simulink model "imageSendExample2"  (R2014a)
settings: configuration reference "AR_Drone_ConfigSet" (kept outside this file)
undefined symbols (not defined in the file or in its folder): Afilter, Afilterphi, Amat, Bd, KDphi, KDphi_adjust, KDpsic, KDtheta, KDtheta_adjust, KDxc, KDyc, KDzc, KPphi, KPphi_adjust, KPpsic, KPtheta, KPtheta_adjust, KPxc, KPyc, KPzc, L, LA, LAphi, m
libraries: simulink x8, dspmtrx3 x5, AR_Drone_2_Library x4, dspstat3 x2, ARdrone_video_lib x1
(part 1 of 2)
settings Model: SimulationMode=external  Creator=Catarina  LastModifiedBy=Catarina

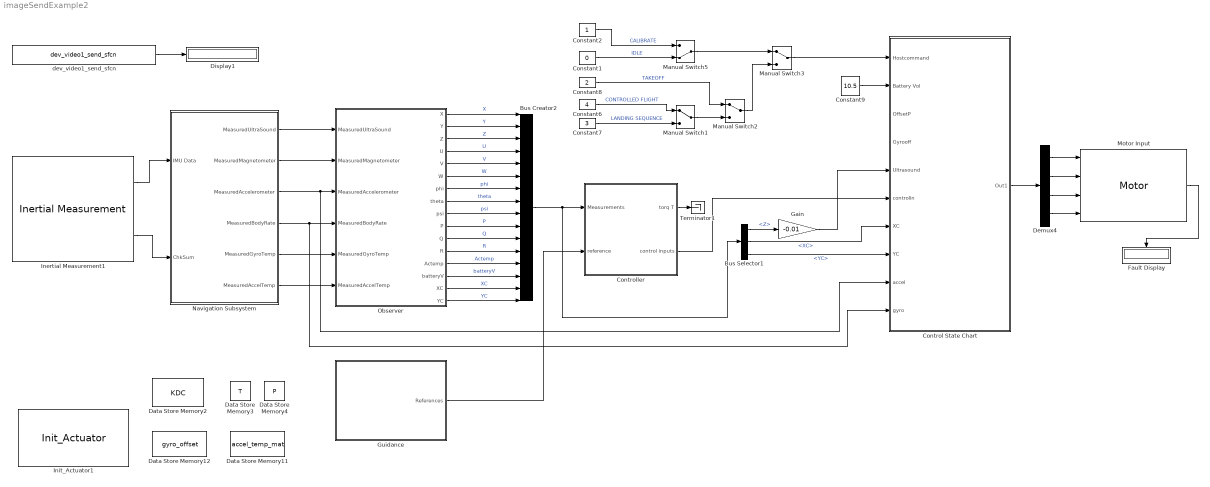
== system imageSendExample2 ==
  Bus Creator2 : BusCreator  Inputs='X','Y','Z','U','V','W','phi','theta','psi','P','Q','R','Actemp','batteryV','XC','YC'
  Bus Selector1 : BusSelector  OutputSignals=Z,XC,YC
  Constant1 : Constant  Value=0
  Constant2 : Constant
  Constant6 : Constant  Value=4
  Constant7 : Constant  Value=3
  Constant8 : Constant  Value=2
  Constant9 : Constant  Value=10.5
  Control State Chart : Subsystem
  Controller : Subsystem
  Data Store Memory11 : DataStoreMemory  DataStoreName=accel_temp_mat  ReadBeforeWriteMsg=warning  WriteAfterWriteMsg=warning  WriteAfterReadMsg=warning  InitialValue=[0 0 0; 0 0 0; 0 0 0]  OutDataTypeStr=double
  Data Store Memory12 : DataStoreMemory  DataStoreName=gyro_offset  ReadBeforeWriteMsg=warning  WriteAfterWriteMsg=warning  WriteAfterReadMsg=warning  InitialValue=[0 0 0]  OutDataTypeStr=double
  Data Store Memory2 : DataStoreMemory  DataStoreName=KDC  ReadBeforeWriteMsg=warning  WriteAfterWriteMsg=warning  WriteAfterReadMsg=warning  OutDataTypeStr=double
  Data Store Memory3 : DataStoreMemory  DataStoreName=T  ReadBeforeWriteMsg=warning  WriteAfterWriteMsg=warning  WriteAfterReadMsg=warning  OutDataTypeStr=double
  Data Store Memory4 : DataStoreMemory  DataStoreName=P  ReadBeforeWriteMsg=warning  WriteAfterWriteMsg=warning  WriteAfterReadMsg=warning  OutDataTypeStr=double
  Demux4 : Demux
  Display1 : Display
  Fault Display : Display
  Gain : Gain  Gain=-0.01
  Guidance : Subsystem
  Inertial Measurement1 : AR_Drone_2_Library/Inertial Measurement  Ts=1/400
  Init_Actuator1 : AR_Drone_2_Library/Init_Actuator  ShowSpec=on
  Manual Switch1 : ManualSwitch
  Manual Switch2 : ManualSwitch
  Manual Switch3 : ManualSwitch
  Manual Switch5 : ManualSwitch  CurrentSetting=0
  Motor Input : AR_Drone_2_Library/Motor
  Navigation Subsystem : Subsystem
  Observer : Subsystem
  Terminator1 : Terminator
  dev_video1_send_sfcn : ARdrone_video_lib/dev_video1_send_sfcn  SFunctionSpec=double y1 = video1GrabSend(int32 work1[1])  SParameter1=[25400]  SParameter2=4  SParameter3=1  SampleTime=1/20  ShowSpec=on
  wires:
  dev_video1_send_sfcn/1 -> Display1/1
  Guidance/1(References) -> Controller/2(reference)
  Constant6/1 -> Manual Switch1/1  "CONTROLLED FLIGHT"
  Constant7/1 -> Manual Switch1/2  "LANDING SEQUENCE"
  Constant8/1 -> Manual Switch2/1  "TAKEOFF"
  Manual Switch1/1 -> Manual Switch2/2
  Constant9/1 -> Control State Chart/2(Battery Vol)
  Controller/2(control inputs) -> Control State Chart/6(controlin)
  Bus Selector1/1 -> Gain/1  "<Z>"
  Bus Selector1/2 -> Control State Chart/7(XC)  "<XC>"
  Bus Selector1/3 -> Control State Chart/8(YC)  "<YC>"
  Gain/1 -> Control State Chart/5(Ultrasound)
  Motor Input/1 -> Fault Display/1
  Demux4/1 -> Motor Input/1
  Demux4/3 -> Motor Input/3
  Control State Chart/1(Out1) -> Demux4/1
  Demux4/4 -> Motor Input/4
  Demux4/2 -> Motor Input/2
  Bus Creator2/1 -> Bus Selector1/1, Controller/1(Measurements)
  Manual Switch2/1 -> Manual Switch3/2
  Inertial Measurement1/1 -> Navigation Subsystem/1(IMU Data)
  Navigation Subsystem/1(MeasuredUltraSound) -> Observer/1(MeasuredUltraSound)
  Navigation Subsystem/2(MeasuredMagnetometer) -> Observer/2(MeasuredMagnetometer)
  Navigation Subsystem/3(MeasuredAccelerometer) -> Control State Chart/9(accel), Observer/3(MeasuredAccelerometer)
  Navigation Subsystem/4(MeasuredBodyRate) -> Control State Chart/10(gyro), Observer/4(MeasuredBodyRate)
  Navigation Subsystem/5(MeasuredGyroTemp) -> Observer/5(MeasuredGyroTemp)
  Navigation Subsystem/6(MeasuredAccelTemp) -> Observer/6(MeasuredAccelTemp)
  Observer/1(X) -> Bus Creator2/1  "X"
  Observer/2(Y) -> Bus Creator2/2  "Y"
  Observer/5(V) -> Bus Creator2/5  "V"
  Observer/4(U) -> Bus Creator2/4  "U"
  Observer/3(Z) -> Bus Creator2/3  "Z"
  Observer/9(psi) -> Bus Creator2/9  "psi"
  Observer/8(theta) -> Bus Creator2/8  "theta"
  Observer/6(W) -> Bus Creator2/6  "W"
  Observer/16(YC) -> Bus Creator2/16  "YC"
  Observer/15(XC) -> Bus Creator2/15  "XC"
  Observer/14(batteryV) -> Bus Creator2/14  "batteryV"
  Observer/13(Actemp) -> Bus Creator2/13  "Actemp"
  Observer/12(R) -> Bus Creator2/12  "R"
  Observer/11(Q) -> Bus Creator2/11  "Q"
  Observer/10(P) -> Bus Creator2/10  "P"
  Observer/7(phi) -> Bus Creator2/7  "phi"
  Manual Switch3/1 -> Control State Chart/1(Hostcommand)
  Constant1/1 -> Manual Switch5/2  "IDLE"
  Constant2/1 -> Manual Switch5/1  "CALIBRATE"
  Manual Switch5/1 -> Manual Switch3/1
  Inertial Measurement1/2 -> Navigation Subsystem/2(ChkSum)
  Controller/1(torq T) -> Terminator1/1

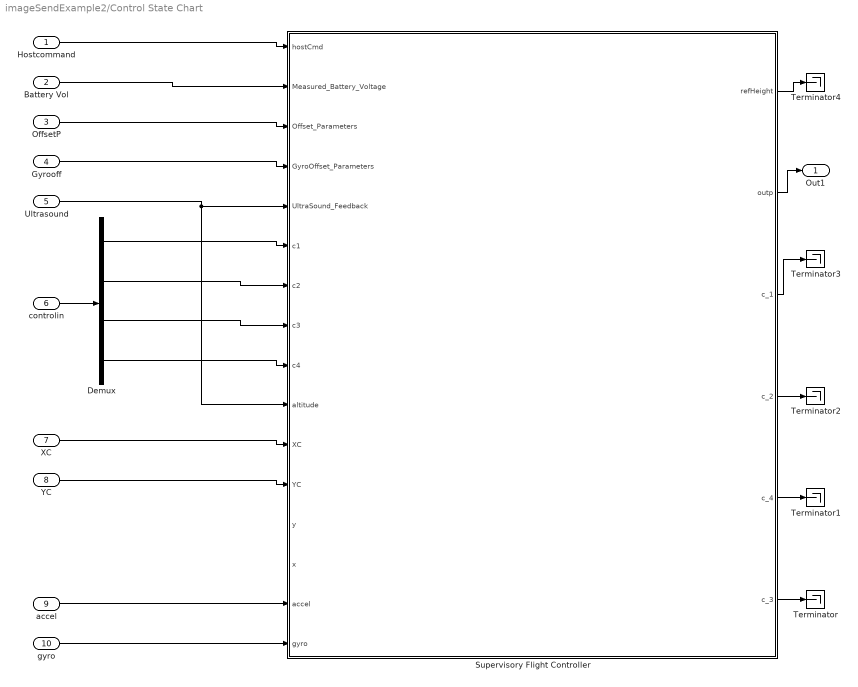
== system imageSendExample2/Control State Chart ==
  Hostcommand : Inport
  Battery Vol : Inport  Port=2
  OffsetP : Inport  Port=3
  Gyrooff : Inport  Port=4
  Ultrasound : Inport  Port=5
  controlin : Inport  Port=6
  XC : Inport  Port=7
  YC : Inport  Port=8
  accel : Inport  Port=9
  gyro : Inport  Port=10
  Demux : Demux
  Supervisory Flight Controller : Stateflow chart  Priority=1  TreatAsAtomicUnit=on
  Terminator{,1..4} (5 alike) : Terminator
  Out1 : Outport
  wires:
  Hostcommand/1 -> Supervisory Flight Controller/1(hostCmd)
  OffsetP/1 -> Supervisory Flight Controller/3(Offset_Parameters)
  Gyrooff/1 -> Supervisory Flight Controller/4(GyroOffset_Parameters)
  Ultrasound/1 -> Supervisory Flight Controller/10(altitude), Supervisory Flight Controller/5(UltraSound_Feedback)
  controlin/1 -> Demux/1
  Battery Vol/1 -> Supervisory Flight Controller/2(Measured_Battery_Voltage)
  Supervisory Flight Controller/2(outp) -> Out1/1
  Demux/1 -> Supervisory Flight Controller/6(c1)
  Demux/2 -> Supervisory Flight Controller/7(c2)
  Demux/3 -> Supervisory Flight Controller/8(c3)
  Demux/4 -> Supervisory Flight Controller/9(c4)
  Supervisory Flight Controller/6(c_3) -> Terminator/1
  Supervisory Flight Controller/3(c_1) -> Terminator3/1
  Supervisory Flight Controller/4(c_2) -> Terminator2/1
  Supervisory Flight Controller/5(c_4) -> Terminator1/1
  Supervisory Flight Controller/1(refHeight) -> Terminator4/1
  XC/1 -> Supervisory Flight Controller/11(XC)
  YC/1 -> Supervisory Flight Controller/12(YC)
  accel/1 -> Supervisory Flight Controller/15(accel)
  gyro/1 -> Supervisory Flight Controller/16(gyro)

== system imageSendExample2/Controller ==
  Measurements : Inport
  reference : Inport  Port=2
  Bus Selector : BusSelector  OutputSignals=X,Y,Z,U,V,W,phi,theta,psi,P,Q,R  OutputAsBus=on
  Control : Subsystem
  Conversion torques to motor speeds : Subsystem
  Mux : Mux
  torq T : Outport
  control inputs : Outport  Port=2
  wires:
  Bus Selector/1 -> Control/1(state)
  Measurements/1 -> Bus Selector/1
  Mux/1 -> Conversion torques to motor speeds/1(torques and thrust), torq T/1
  Control/2(torquephi) -> Mux/2
  Control/3(torquetheta) -> Mux/3
  Control/4(torquepsi) -> Mux/4
  reference/1 -> Control/2(reference)
  Control/1(thrust) -> Mux/1
  Conversion torques to motor speeds/1(Motor speeds) -> control inputs/1

== system imageSendExample2/Guidance ==
  Constant : Constant  Value=0
  Constant1 : Constant  Value=0
  Constant2 : Constant  Value=0
  Data Store Read : DataStoreRead  DataStoreName=KDC
  Gain : Gain  Gain=-1
  Mux2 : Mux  Inputs=16
  References : Outport
  wires:
  Mux2/1 -> References/1
  Constant/1 -> Mux2/9, Mux2/10, Mux2/11, Mux2/12, Mux2/14, Mux2/15, Mux2/16, Mux2/13, Mux2/6, Mux2/5, Mux2/1, Mux2/4
  Constant1/1 -> Mux2/2
  Constant2/1 -> Mux2/8, Mux2/7
  Data Store Read/1 -> Gain/1
  Gain/1 -> Mux2/3

== system imageSendExample2/Navigation Subsystem ==
  IMU Data : Inport
  ChkSum : Inport  Port=2
  CheckSum Pre-Processing : Subsystem
  MeasuredUltraSound : Outport
  MeasuredMagnetometer : Outport  Port=2
  MeasuredAccelerometer : Outport  Port=3
  MeasuredBodyRate : Outport  Port=4
  MeasuredGyroTemp : Outport  Port=5
  MeasuredAccelTemp : Outport  Port=6
  wires:
  IMU Data/1 -> CheckSum Pre-Processing/1(IMU Packets)
  ChkSum/1 -> CheckSum Pre-Processing/2(CheckSumFlag)
  CheckSum Pre-Processing/1(UltraSoundHeight_Processed) -> MeasuredUltraSound/1
  CheckSum Pre-Processing/4(Accelerometer) -> MeasuredAccelerometer/1
  CheckSum Pre-Processing/3(Body Rates - pqr) -> MeasuredBodyRate/1
  CheckSum Pre-Processing/2(Magnetometer_Processed) -> MeasuredMagnetometer/1
  CheckSum Pre-Processing/5(TempMeasure) -> MeasuredGyroTemp/1
  CheckSum Pre-Processing/6(AccelTempMeasure) -> MeasuredAccelTemp/1

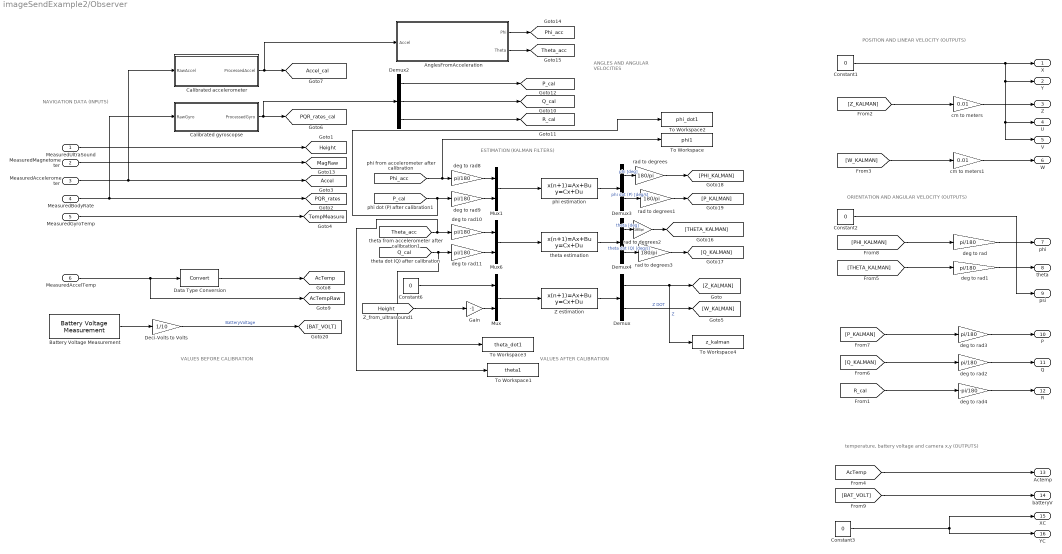
== system imageSendExample2/Observer ==
  note: temperature, battery voltage and camera x,y (OUTPUTS)
  note: ORIENTATION AND ANGULAR VELOCITY (OUTPUTS)
  note: POSITION AND LINEAR VELOCITY (OUTPUTS)
  note: NAVIGATION
      | DATA
      | (INPUTS)
  note: ESTIMATION (KALMAN FILTERS)
  note: ANGLES AND
      | ANGULAR
      | VELOCITIES
  note: VALUES BEFORE CALIBRATION
  note: VALUES AFTER CALIBRATION
  MeasuredUltraSound : Inport
  MeasuredMagnetometer : Inport  Port=2
  MeasuredAccelerometer : Inport  Port=3
  MeasuredBodyRate : Inport  Port=4
  MeasuredGyroTemp : Inport  Port=5
  MeasuredAccelTemp : Inport  Port=6
  AnglesFromAcceleration : Subsystem
  Battery Voltage Measurement : AR_Drone_2_Library/Battery Voltage Measurement  SFunctionSpec=void BatteryMeasure_step(single y1[1])  SampleTime=-1
  Calibrated accelerometer : Subsystem
  Calibrated gyroscopse : Subsystem
  Constant{1..3,6} (4 alike) : Constant  Value=0
  Data Type Conversion : DataTypeConversion
  Deci-Volts to Volts : Gain  Gain=1/10
  Demux : Demux  Outputs=2
  Demux2 : Demux  Outputs=3
  Demux3 : Demux  Outputs=2
  Demux4 : Demux  Outputs=2
  Gain : Gain  Gain=-1
  Mux : Mux  Inputs=2
  Mux1 : Mux  Inputs=2
  Mux6 : Mux  Inputs=2
  To Workspace : ToWorkspace  VariableName=phi1  SaveFormat=Structure With Time  SampleTime=-1
  To Workspace1 : ToWorkspace  VariableName=theta1  SaveFormat=Structure With Time  SampleTime=-1
  To Workspace2 : ToWorkspace  VariableName=phi_dot1  SaveFormat=Structure With Time  SampleTime=-1
  To Workspace3 : ToWorkspace  VariableName=theta_dot1  SaveFormat=Structure With Time  SampleTime=-1
  To Workspace4 : ToWorkspace  VariableName=z_kalman  SaveFormat=Structure With Time  SampleTime=-1
  Z estimation : DiscreteStateSpace  A=Amat  B=[Bd L]  C=eye(2)  D=zeros(2)  X0=[0,0]  SampleTime=-1
  cm to meters : Gain  Gain=0.01
  cm to meters1 : Gain  Gain=0.01
  deg to rad{,1..3,8..11} (8 alike) : Gain  Gain=pi/180
  deg to rad4 : Gain  Gain=-pi/180
  phi estimation : DiscreteStateSpace  A=Afilterphi  B=[LAphi]  C=eye(2)  D=zeros(2)  X0=[0,0]  SampleTime=-1
  rad to degrees{,1..3} (4 alike) : Gain  Gain=180/pi
  theta estimation : DiscreteStateSpace  A=Afilter  B=[LA]  C=eye(2)  D=zeros(2)  X0=[0,0]  SampleTime=-1
  X : Outport
  Y : Outport  Port=2
  Z : Outport  Port=3
  U : Outport  Port=4
  V : Outport  Port=5
  W : Outport  Port=6
  phi : Outport  Port=7
  theta : Outport  Port=8
  psi : Outport  Port=9
  P : Outport  Port=10
  Q : Outport  Port=11
  R : Outport  Port=12
  Actemp : Outport  Port=13
  batteryV : Outport  Port=14
  XC : Outport  Port=15
  YC : Outport  Port=16
  tag scope: AcTemp=global, AcTempRaw=global, Accel=global, Accel_cal=global, Height=global, MagRaw=global, PQR_rates=global, PQR_rates_cal=global, P_cal=global, Phi_acc=global, Q_cal=global, R_cal=global, TempMeasure=global, Theta_acc=global
  wires:
  Mux1/1 -> phi estimation/1
  phi estimation/1 -> Demux3/1
  Battery Voltage Measurement/1 -> Deci-Volts to Volts/1
  MeasuredMagnetometer/1 -> [MagRaw]
  MeasuredAccelerometer/1 -> Calibrated accelerometer/1(RawAccel), [Accel]
  MeasuredGyroTemp/1 -> [TempMeasure]
  MeasuredUltraSound/1 -> [Height]
  Mux6/1 -> theta estimation/1
  theta estimation/1 -> Demux4/1
  Z estimation/1 -> Demux/1
  Constant6/1 -> Mux/1
  Demux/2 -> [W_KALMAN]  "Z DOT"
  Demux/1 -> To Workspace4/1, [Z_KALMAN]  "Z"
  Gain/1 -> Mux/2
  Mux/1 -> Z estimation/1
  [Height] -> Gain/1
  Data Type Conversion/1 -> [AcTemp]
  MeasuredAccelTemp/1 -> [AcTempRaw], Data Type Conversion/1
  Calibrated accelerometer/1(ProcessedAccel) -> [Accel_cal], AnglesFromAcceleration/1(Accel)
  Demux2/2 -> [Q_cal]
  Calibrated gyroscopse/1(ProcessedGyro) -> [PQR_rates_cal], Demux2/1
  Demux2/1 -> [P_cal]
  Demux2/3 -> [R_cal]
  AnglesFromAcceleration/1(Phi) -> [Phi_acc]
  AnglesFromAcceleration/2(Theta) -> [Theta_acc]
  [P_cal] -> To Workspace2/1, deg to rad9/1
  [Q_cal] -> To Workspace3/1, deg to rad11/1
  [Phi_acc] -> To Workspace/1, deg to rad8/1
  Constant1/1 -> V/1, U/1, Y/1, X/1
  [Z_KALMAN] -> cm to meters/1
  [AcTemp] -> Actemp/1
  deg to rad/1 -> phi/1
  cm to meters/1 -> Z/1
  [THETA_KALMAN] -> deg to rad1/1
  [Q_KALMAN] -> deg to rad2/1
  [P_KALMAN] -> deg to rad3/1
  [PHI_KALMAN] -> deg to rad/1
  [BAT_VOLT] -> batteryV/1
  cm to meters1/1 -> W/1
  [W_KALMAN] -> cm to meters1/1
  deg to rad1/1 -> theta/1
  deg to rad3/1 -> P/1
  deg to rad2/1 -> Q/1
  Constant2/1 -> psi/1
  Constant3/1 -> XC/1, YC/1
  Demux4/2 -> rad to degrees3/1  "theta dot (Q) [deg/s]"
  Demux3/1 -> rad to degrees/1  "phi [deg]"
  Demux3/2 -> rad to degrees1/1  "phi dot (P) [deg/s]"
  Demux4/1 -> rad to degrees2/1  "theta [deg]"
  Deci-Volts to Volts/1 -> [BAT_VOLT]  "BatteryVoltage"
  [Theta_acc] -> To Workspace1/1, deg to rad10/1
  deg to rad8/1 -> Mux1/1
  deg to rad9/1 -> Mux1/2
  deg to rad10/1 -> Mux6/1
  deg to rad11/1 -> Mux6/2
  rad to degrees/1 -> [PHI_KALMAN]
  rad to degrees1/1 -> [P_KALMAN]
  rad to degrees2/1 -> [THETA_KALMAN]
  rad to degrees3/1 -> [Q_KALMAN]
  MeasuredBodyRate/1 -> [PQR_rates], Calibrated gyroscopse/1(RawGyro)
  [R_cal] -> deg to rad4/1
  deg to rad4/1 -> R/1

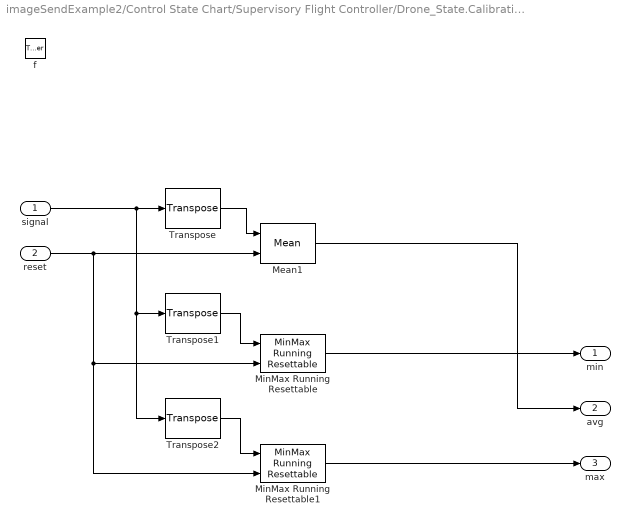
== system imageSendExample2/Control State Chart/Supervisory Flight Controller/Drone_State.Calibration.calibAccel ==
  signal : Inport  OutDataTypeStr=double  PortDimensions=3
  reset : Inport  Port=2  OutDataTypeStr=double  PortDimensions=1
  f : TriggerPort  TriggerType=function-call
      settings: CopyFcn=Stateflow.SLINSF.SimulinkMan.removeBlockPreDeleteFcn  PreDeleteFcn=Stateflow.SLINSF.SimulinkMan.unsafePredeleteFcn
  Mean1 : dspstat3/Mean  run=on  reset_popup=Non-zero sample  InputProcessing=Columns as channels (frame based)  directionMode=Entire input  dimension=1  treatSBRowAsCol=on  roiEnable=off  roiType=Rectangles  roiPortion=Entire ROI  roiOutput=Individual statistics for each ROI  roiFlag=off  outputDataTypeStr=Inherit: Same as accumulator  outputLastDataTypeStr=Inherit: Same as accumulator  outputMin=[]  outputMax=[]  roundingMode=Nearest  overflowMode=off
  MinMax Running Resettable : simulink/Math Operations/MinMax Running Resettable  Function=min  vinit=inf
  MinMax Running Resettable1 : simulink/Math Operations/MinMax Running Resettable  Function=max  vinit=-inf
  Transpose : dspmtrx3/Transpose  Hermitian=off  overflowFlag=off
  Transpose1 : dspmtrx3/Transpose  Hermitian=off  overflowFlag=off
  Transpose2 : dspmtrx3/Transpose  Hermitian=off  overflowFlag=off
  min : Outport
  avg : Outport  Port=2
  max : Outport  Port=3
  wires:
  signal/1 -> Transpose2/1, Transpose1/1, Transpose/1
  Mean1/1 -> avg/1
  Transpose/1 -> Mean1/1
  reset/1 -> MinMax Running Resettable1/2, MinMax Running Resettable/2, Mean1/2
  MinMax Running Resettable1/1 -> max/1
  MinMax Running Resettable/1 -> min/1
  Transpose1/1 -> MinMax Running Resettable/1
  Transpose2/1 -> MinMax Running Resettable1/1

== system imageSendExample2/Control State Chart/Supervisory Flight Controller/Drone_State.Calibration.calibGyro ==
  signal : Inport  OutDataTypeStr=double  PortDimensions=3
  reset : Inport  Port=2  OutDataTypeStr=double  PortDimensions=1
  f : TriggerPort  TriggerType=function-call
      settings: CopyFcn=Stateflow.SLINSF.SimulinkMan.removeBlockPreDeleteFcn  PreDeleteFcn=Stateflow.SLINSF.SimulinkMan.unsafePredeleteFcn
  Mean1 : dspstat3/Mean  run=on  reset_popup=Non-zero sample  InputProcessing=Columns as channels (frame based)  directionMode=Entire input  dimension=1  treatSBRowAsCol=on  roiEnable=off  roiType=Rectangles  roiPortion=Entire ROI  roiOutput=Individual statistics for each ROI  roiFlag=off  outputDataTypeStr=Inherit: Same as accumulator  outputLastDataTypeStr=Inherit: Same as accumulator  outputMin=[]  outputMax=[]  roundingMode=Nearest  overflowMode=off
  Transpose : dspmtrx3/Transpose  Hermitian=off  overflowFlag=off
  gyro : Outport
  wires:
  signal/1 -> Transpose/1
  Mean1/1 -> gyro/1
  Transpose/1 -> Mean1/1
  reset/1 -> Mean1/2

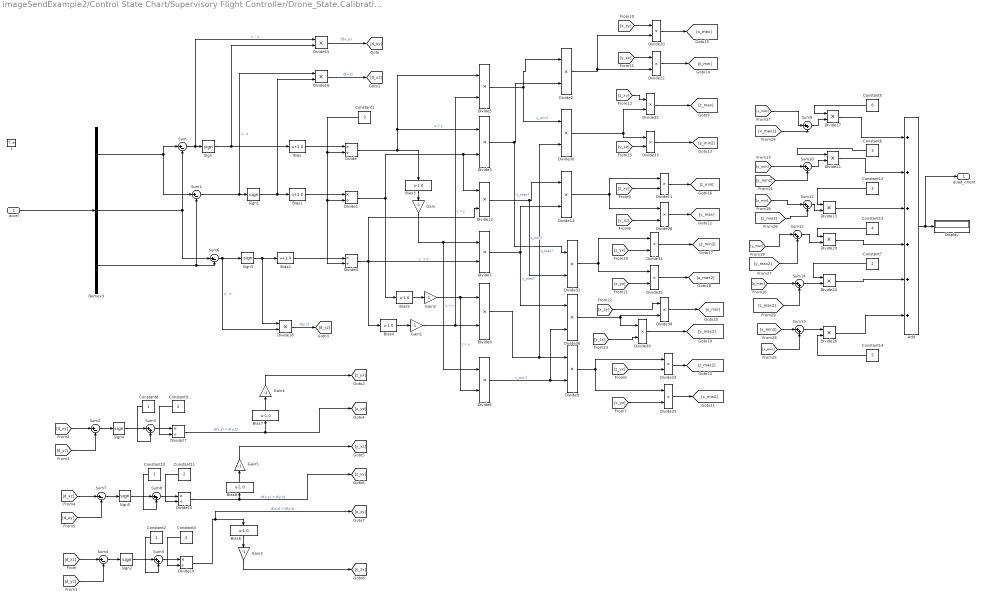
== system imageSendExample2/Control State Chart/Supervisory Flight Controller/Drone_State.Calibration.getPosition ==
  note: d(x,y)
  accel : Inport  OutDataTypeStr=double  PortDimensions=3
  f : TriggerPort  TriggerType=function-call
      settings: CopyFcn=Stateflow.SLINSF.SimulinkMan.removeBlockPreDeleteFcn  PreDeleteFcn=Stateflow.SLINSF.SimulinkMan.unsafePredeleteFcn
  Add : Sum  Inputs=++++++
  Bias : Bias  Bias=1.0
  Bias1 : Bias  Bias=1.0
  Bias2 : Bias  Bias=1.0
  Bias{3..8} (6 alike) : Bias  Bias=-1.0
  Constant{1,3,7,9,11} (5 alike) : Constant  Value=2
  Constant{2,8,10,12} (4 alike) : Constant
  Constant13 : Constant  Value=4
  Constant14 : Constant  Value=5
  Constant5 : Constant  Value=6
  Constant6 : Constant  Value=3
  Demux3 : Demux  Outputs=3
  Display : Display
  Divide{,1,4,10,19,27} (6 alike) : Product  Inputs=*/
  Divide{2..3,5..9,11..18,20..26,28..36,38..39} (33 alike) : Product  Inputs=**
  Gain{,1..5} (6 alike) : Gain  Gain=-1
  Sign{,1..5} (6 alike) : Signum
  Sum{,1..2,4,6..7} (6 alike) : Sum  Inputs=|+-
  Sum{3,5,8..14} (9 alike) : Sum  Inputs=|++
  quad_orient : Outport  OutDataTypeStr=double  PortDimensions=1
  wires:
  Demux3/3 -> Sum1/2, Sum6/2
  Demux3/1 -> Sum/1, Sum1/1
  Constant1/1 -> Divide/2, Divide1/2, Divide4/2
  Bias1/1 -> Divide1/1
  Divide/1 -> Bias3/1, Divide3/1, Divide5/1  "x > y"
  Divide1/1 -> Divide12/1, Divide3/2, Bias5/1
  Sum6/1 -> Sign3/1, Divide18/2  "y - z"
  Demux3/2 -> Sum/2, Sum6/1
  Sign3/1 -> Bias2/1, Divide18/1
  Bias2/1 -> Divide4/1
  Divide4/1 -> Bias4/1, Divide7/2, Divide12/2  "y  > z"
  Bias3/1 -> Gain/1
  Gain/1 -> Divide6/1, Divide7/1  "y > x"
  Bias4/1 -> Gain1/1
  Gain1/1 -> Divide5/2, Divide8/2  "z > y"
  Bias5/1 -> Gain2/1
  Gain2/1 -> Divide6/2, Divide8/1  "z > x"
  Divide3/1 -> Divide31/1, Divide2/2  "x_max?"
  Divide5/1 -> Divide2/1, Divide30/1  "y_min?"
  Divide6/1 -> Divide36/2, Divide9/2  "x_min?"
  Divide8/1 -> Divide30/2, Divide9/1  "z_max?"
  Divide7/1 -> Divide36/1, Divide14/2  "y_max?"
  Divide12/1 -> Divide14/1, Divide31/2  "z_min?"
  Divide18/1 -> [d_yz]  "d(y,z)"
  Bias/1 -> Divide/1
  Sum/1 -> Divide15/1, Sign/1  "x  - y"
  Sum1/1 -> Divide16/1, Sign1/1  "x - z"
  Sign/1 -> Divide15/2, Bias/1
  Sign1/1 -> Divide16/2, Bias1/1
  Divide15/1 -> [d_xy]
  Divide16/1 -> [d_xz]  "d(x,z)"
  [d_xy] -> Sum2/1
  [d_yz] -> Sum2/2
  Sum2/1 -> Sign4/1
  Sign4/1 -> Sum3/1
  Constant8/1 -> Sum3/2
  Sum3/1 -> Divide27/1
  Constant9/1 -> Divide27/2
  Divide27/1 -> [x_yz], Bias7/1  "d(x,y) > d(y,z)"
  Bias7/1 -> Gain4/1
  Gain4/1 -> [z_yx]
  [d_xz] -> Sum7/1
  [d_xy] -> Sum7/2
  Sum7/1 -> Sign5/1
  Sign5/1 -> Sum8/1
  Constant10/1 -> Sum8/2
  Sum8/1 -> Divide10/1
  Constant11/1 -> Divide10/2
  Bias8/1 -> Gain5/1
  Divide10/1 -> Bias8/1, [z_xy]  "d(x,y) > d(y,z)"
  Gain5/1 -> [y_xz]
  [d_xz] -> Sum4/1
  [d_yz] -> Sum4/2
  Sum4/1 -> Sign2/1
  Sign2/1 -> Sum5/1
  Constant2/1 -> Sum5/2
  Sum5/1 -> Divide19/1
  Constant3/1 -> Divide19/2
  Bias6/1 -> Gain3/1
  Divide19/1 -> Bias6/1, [x_zy]  "d(x,z) > d(y,z)"
  Gain3/1 -> [y_zx]
  Divide2/1 -> Divide20/2, Divide22/2
  [x_zy] -> Divide20/1
  [y_zx] -> Divide22/1
  [z_xy] -> Divide32/1
  Divide30/1 -> Divide32/2, Divide33/1
  Divide32/1 -> [z_max]
  Divide33/1 -> [y_min2]
  [y_xz] -> Divide33/2
  Divide22/1 -> [y_min]
  Divide20/1 -> [x_max]
  Divide14/1 -> Divide11/1, Divide28/1
  [y_xz] -> Divide28/2
  [z_xy] -> Divide11/2
  Divide28/1 -> [y_max]
  Divide11/1 -> [z_min]
  [z_yx] -> Divide34/2
  Divide31/1 -> Divide34/1, Divide35/1
  Divide34/1 -> [z_min2]
  [x_yz] -> Divide35/2
  Divide35/1 -> [x_max2]
  Divide9/1 -> Divide23/1, Divide25/1
  [z_yx] -> Divide23/2
  [x_yz] -> Divide25/2
  Divide23/1 -> [z_max2]
  Divide25/1 -> [x_min2]
  [y_zx] -> Divide39/2
  Divide39/1 -> [y_max2]
  Divide36/1 -> Divide39/1, Divide38/2
  [x_zy] -> Divide38/1
  Divide38/1 -> [x_min]
  Constant5/1 -> Divide17/1
  Constant6/1 -> Divide21/1
  Constant7/1 -> Divide24/1
  Constant13/1 -> Divide29/1
  Divide17/1 -> Add/1
  Divide21/1 -> Add/2
  Add/1 -> quad_orient/1, Display/1
  Divide13/1 -> Add/3
  Divide29/1 -> Add/4
  Divide24/1 -> Add/5
  Divide26/1 -> Add/6
  Sum9/1 -> Divide17/2
  [x_max] -> Sum9/1
  [x_max2] -> Sum9/2
  Sum10/1 -> Divide21/2
  [y_min2] -> Sum10/2
  Constant12/1 -> Divide13/1
  Sum11/1 -> Divide13/2
  [z_min2] -> Sum11/2
  Sum12/1 -> Divide29/2
  [y_max2] -> Sum12/2
  [x_min2] -> Sum13/1
  Sum13/1 -> Divide26/1
  Constant14/1 -> Divide26/2
  [x_min] -> Sum13/2
  Sum14/1 -> Divide24/2
  [z_max] -> Sum14/1
  [z_max2] -> Sum14/2
  [y_min] -> Sum10/1
  [z_min] -> Sum11/1
  [y_max] -> Sum12/1
  accel/1 -> Demux3/1

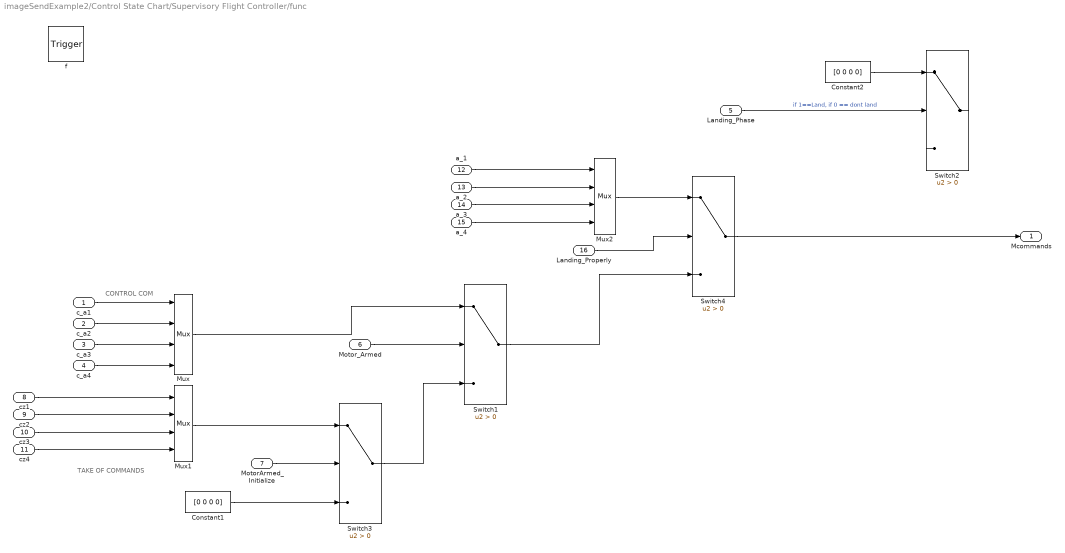
== system imageSendExample2/Control State Chart/Supervisory Flight Controller/func ==
  note: CONTROL COM
  note: TAKE OF COMMANDS
  c_a1 : Inport  OutDataTypeStr=double  PortDimensions=1
  c_a2 : Inport  Port=2  OutDataTypeStr=double  PortDimensions=1
  c_a3 : Inport  Port=3  OutDataTypeStr=double  PortDimensions=1
  c_a4 : Inport  Port=4  OutDataTypeStr=double  PortDimensions=1
  Landing_Phase : Inport  Port=5  OutDataTypeStr=double  PortDimensions=1
  Motor_Armed : Inport  Port=6  OutDataTypeStr=double  PortDimensions=1
  MotorArmed_Initialize : Inport  Port=7  OutDataTypeStr=double  PortDimensions=1
  cz1 : Inport  Port=8  OutDataTypeStr=double  PortDimensions=1
  cz2 : Inport  Port=9  OutDataTypeStr=double  PortDimensions=1
  cz3 : Inport  Port=10  OutDataTypeStr=double  PortDimensions=1
  cz4 : Inport  Port=11  OutDataTypeStr=double  PortDimensions=1
  a_1 : Inport  Port=12  OutDataTypeStr=double  PortDimensions=1
  a_2 : Inport  Port=13  OutDataTypeStr=double  PortDimensions=1
  a_3 : Inport  Port=14  OutDataTypeStr=double  PortDimensions=1
  a_4 : Inport  Port=15  OutDataTypeStr=double  PortDimensions=1
  Landing_Properly : Inport  Port=16  OutDataTypeStr=double  PortDimensions=1
  f : TriggerPort  TriggerType=function-call
      settings: CopyFcn=Stateflow.SLINSF.SimulinkMan.removeBlockPreDeleteFcn  PreDeleteFcn=Stateflow.SLINSF.SimulinkMan.unsafePredeleteFcn
  Constant1 : Constant  Value=[0 0 0 0]  OutDataTypeStr=int16
  Constant2 : Constant  Value=[0 0 0 0]  OutDataTypeStr=int16
  Mux : Mux
  Mux1 : Mux
  Mux2 : Mux
  Switch{1..4} (4 alike) : Switch  Criteria=u2 > Threshold
  Mcommands : Outport
  wires:
  Motor_Armed/1 -> Switch1/2
  Mux/1 -> Switch1/1
  c_a1/1 -> Mux/1
  c_a2/1 -> Mux/2
  c_a3/1 -> Mux/3
  c_a4/1 -> Mux/4
  Landing_Phase/1 -> Switch2/2  "if 1==Land, if 0 == dont land"
  Constant2/1 -> Switch2/1
  MotorArmed_Initialize/1 -> Switch3/2
  cz1/1 -> Mux1/1
  cz2/1 -> Mux1/2
  cz3/1 -> Mux1/3
  Switch3/1 -> Switch1/3
  Mux1/1 -> Switch3/1
  Constant1/1 -> Switch3/3
  a_1/1 -> Mux2/1
  a_2/1 -> Mux2/2
  a_3/1 -> Mux2/3
  a_4/1 -> Mux2/4
  Mux2/1 -> Switch4/1
  Landing_Properly/1 -> Switch4/2
  Switch1/1 -> Switch4/3
  Switch4/1 -> Mcommands/1
  cz4/1 -> Mux1/4

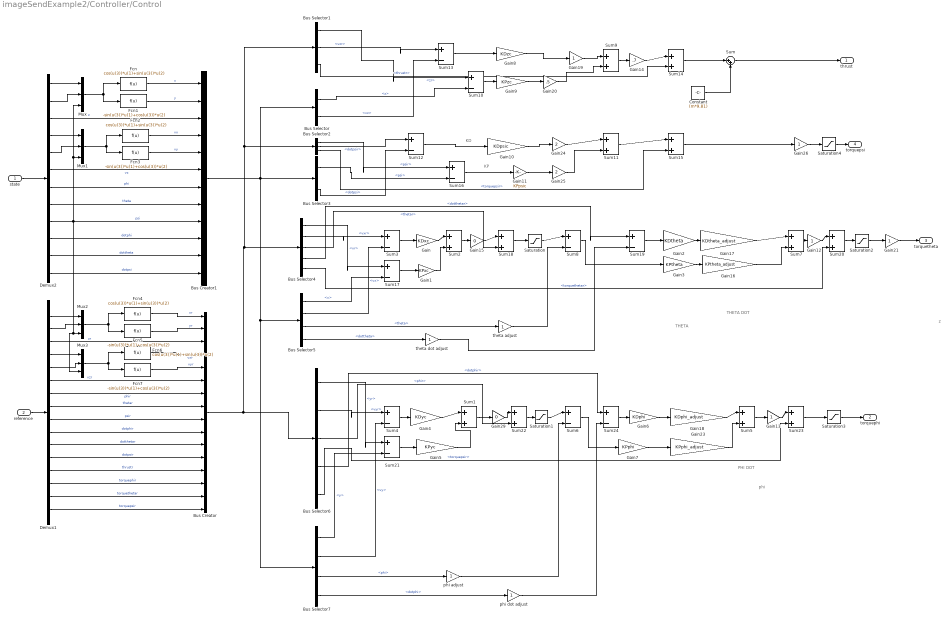
== system imageSendExample2/Controller/Control ==
  note: KP
  note: KD
  note: z
  note: PHI DOT
  note: phi
  note: THETA DOT
  note: THETA
  state : Inport
  reference : Inport  Port=2
  Bus Creator : BusCreator  Inputs='xr','yr','zr','vxr','vyr','vzr','phir','thetar','psir','dotphir','dotthetar','dotpsir','thrustr','torquephir','torquethetar','torquepsir'
  Bus Creator1 : BusCreator  Inputs='x','y','z','vx','vy','vz','phi','theta','psi','dotphi','dottheta','dotpsi'
  Bus Selector : BusSelector  OutputSignals=z,vz
  Bus Selector1 : BusSelector  OutputSignals=zr,vzr,thrustr
  Bus Selector2 : BusSelector  OutputSignals=psir,dotpsir,torquepsir
  Bus Selector3 : BusSelector  OutputSignals=psi,dotpsi
  Bus Selector4 : BusSelector  OutputSignals=xr,vxr,thetar,dotthetar,torquethetar
  Bus Selector5 : BusSelector  OutputSignals=x,vx,theta,dottheta
  Bus Selector6 : BusSelector  OutputSignals=yr,vyr,phir,dotphir,torquepsir
  Bus Selector7 : BusSelector  OutputSignals=y,vy,phi,dotphi
  Constant : Constant  Value=(m*9.81)
  Demux1 : Demux  Outputs=16
  Demux2 : Demux  Outputs=12
  Fcn{,2,4,6} (4 alike) : Fcn  Expr=cos(u(3))*u(1)+sin(u(3))*u(2)
  Fcn{1,3,5,7} (4 alike) : Fcn  Expr=-sin(u(3))*u(1)+cos(u(3))*u(2)
  Gain : Gain  Gain=KDxc
  Gain1 : Gain  Gain=KPxc
  Gain10 : Gain  Gain=KDpsic
  Gain11 : Gain  Gain=KPpsic
  Gain{12..13,19,21,26} (5 alike) : Gain
  Gain14 : Gain  Gain=.7
  Gain15 : Gain  Gain=0
  Gain16 : Gain  Gain=KPtheta_adjust
  Gain17 : Gain  Gain=KDtheta_adjust
  Gain18 : Gain  Gain=KDphi_adjust
  Gain2 : Gain  Gain=KDtheta
  Gain20 : Gain  Gain=.5
  Gain23 : Gain  Gain=KPphi_adjust
  Gain24 : Gain  Gain=2
  Gain25 : Gain  Gain=2
  Gain29 : Gain  Gain=0
  Gain3 : Gain  Gain=KPtheta
  Gain4 : Gain  Gain=KDyc
  Gain5 : Gain  Gain=KPyc
  Gain6 : Gain  Gain=KDphi
  Gain7 : Gain  Gain=KPphi
  Gain8 : Gain  Gain=KDzc
  Gain9 : Gain  Gain=KPzc
  Mux{,1..3} (4 alike) : Mux  Inputs=3
  Saturation{,1..4} (5 alike) : Saturate  UpperLimit=0.8  LowerLimit=-0.8
  Sum{,1..2,5,7,9,11,14..15,18,20,22..23} (13 alike) : Sum  Inputs=|++
  Sum{3..4,6,8,10,12..13,16..17,19,21,24} (12 alike) : Sum  Inputs=|+-
  phi adjust : Gain
  phi dot adjust : Gain
  theta adjust : Gain
  theta dot adjust : Gain
  thrust : Outport
  torquephi : Outport  Port=2
  torquetheta : Outport  Port=3
  torquepsi : Outport  Port=4
  wires:
  Gain/1 -> Sum2/1
  Sum3/1 -> Gain/1
  Gain1/1 -> Sum2/2
  Bus Selector5/2 -> Sum3/2  "<vx>"
  Sum17/1 -> Gain1/1
  Gain5/1 -> Sum1/2
  Gain4/1 -> Sum1/1
  Sum4/1 -> Gain4/1
  Gain7/1 -> Gain23/1
  Gain6/1 -> Gain18/1
  Saturation1/1 -> Sum6/1
  Gain9/1 -> Gain20/1
  Gain8/1 -> Gain19/1
  Sum11/1 -> Sum15/1
  Sum12/1 -> Gain10/1
  Gain10/1 -> Gain24/1
  Gain11/1 -> Gain25/1
  Bus Selector1/1 -> Sum10/1  "<zr>"
  Bus Selector/1 -> Sum10/2  "<z>"
  Sum10/1 -> Gain9/1
  Bus Selector/2 -> Sum13/2  "<vz>"
  Sum13/1 -> Gain8/1
  Bus Selector1/2 -> Sum13/1  "<vzr>"
  Bus Selector1/3 -> Sum14/2  "<thrustr>"
  Sum9/1 -> Gain14/1
  Sum16/1 -> Gain11/1
  Bus Selector2/1 -> Sum16/1  "<psir>"
  Bus Selector2/2 -> Sum12/1  "<dotpsir>"
  Bus Selector2/3 -> Sum15/2  "<torquepsir>"
  Bus Selector5/1 -> Sum17/2  "<x>"
  Bus Selector4/1 -> Sum17/1  "<xr>"
  Bus Selector4/2 -> Sum3/1  "<vxr>"
  Sum2/1 -> Gain15/1
  Sum18/1 -> Saturation/1
  Bus Selector4/3 -> Sum18/2  "<thetar>"
  Bus Selector5/3 -> theta adjust/1  "<theta>"
  Bus Selector5/4 -> theta dot adjust/1  "<dottheta>"
  Bus Selector4/4 -> Sum19/1  "<dotthetar>"
  Sum19/1 -> Gain2/1
  Saturation/1 -> Sum8/1
  Sum20/1 -> Saturation2/1
  Bus Selector4/5 -> Sum20/2  "<torquethetar>"
  Sum21/1 -> Gain5/1
  Sum22/1 -> Saturation1/1
  Sum1/1 -> Gain29/1
  Bus Selector6/3 -> Sum22/2  "<phir>"
  Sum23/1 -> Saturation3/1
  Sum5/1 -> Gain13/1
  Bus Selector6/5 -> Sum23/2  "<torquepsir>"
  Sum24/1 -> Gain6/1
  Bus Selector6/4 -> Sum24/1  "<dotphir>"
  Bus Selector7/4 -> phi dot adjust/1  "<dotphi>"
  Bus Selector6/1 -> Sum21/1  "<yr>"
  Bus Selector6/2 -> Sum4/1  "<vyr>"
  Bus Selector7/2 -> Sum4/2  "<vy>"
  Bus Selector3/1 -> Sum16/2  "<psi>"
  Bus Selector3/2 -> Sum12/2  "<dotpsi>"
  Sum15/1 -> Gain26/1
  Saturation3/1 -> torquephi/1
  Sum14/1 -> Sum/1
  Sum/1 -> thrust/1
  Constant/1 -> Sum/2
  Demux2/3 -> Bus Creator1/3  "z"
  Demux2/6 -> Bus Creator1/6  "vz"
  Demux2/7 -> Bus Creator1/7  "phi"
  Demux2/8 -> Bus Creator1/8  "theta"
  Demux2/9 -> Mux3/3, Mux2/3, Mux1/3, Mux/3, Bus Creator1/9  "psi"
  Demux2/10 -> Bus Creator1/10  "dotphi"
  Demux2/11 -> Bus Creator1/11  "dottheta"
  Demux2/12 -> Bus Creator1/12  "dotpsi"
  state/1 -> Demux2/1
  Bus Creator1/1 -> Bus Selector7/1, Bus Selector5/1, Bus Selector3/1, Bus Selector/1
  Demux1/16 -> Bus Creator/16  "torquepsir"
  Demux1/15 -> Bus Creator/15  "torquethetar"
  Demux1/14 -> Bus Creator/14  "torquephir"
  Demux1/13 -> Bus Creator/13  "thrustr"
  Demux1/12 -> Bus Creator/12  "dotpsir"
  Demux1/11 -> Bus Creator/11  "dotthetar"
  Demux1/10 -> Bus Creator/10  "dotphir"
  Demux1/9 -> Bus Creator/9  "psir"
  Demux1/8 -> Bus Creator/8  "thetar"
  Demux1/7 -> Bus Creator/7  "phir"
  Demux1/6 -> Bus Creator/6  "vzr"
  Demux1/3 -> Bus Creator/3  "zr"
  Bus Creator/1 -> Bus Selector2/1, Bus Selector1/1, Bus Selector4/1, Bus Selector6/1
  reference/1 -> Demux1/1
  Fcn/1 -> Bus Creator1/1  "x"
  Mux/1 -> Fcn/1, Fcn1/1
  Fcn1/1 -> Bus Creator1/2  "y"
  Demux2/1 -> Mux/1
  Demux2/2 -> Mux/2
  Demux2/4 -> Mux1/1
  Demux2/5 -> Mux1/2
  Fcn2/1 -> Bus Creator1/4  "vx"
  Mux1/1 -> Fcn2/1, Fcn3/1
  Fcn3/1 -> Bus Creator1/5  "vy"
  Demux1/1 -> Mux2/1
  Demux1/2 -> Mux2/2
  Demux1/4 -> Mux3/1
  Demux1/5 -> Mux3/2
  Mux2/1 -> Fcn5/1, Fcn4/1
  Fcn5/1 -> Bus Creator/2  "yr"
  Fcn6/1 -> Bus Creator/4  "vxr"
  Mux3/1 -> Fcn7/1, Fcn6/1
  Fcn7/1 -> Bus Creator/5  "vyr"
  Sum7/1 -> Gain12/1
  Gain12/1 -> Sum20/1
  Gain13/1 -> Sum23/1
  Gain14/1 -> Sum14/1
  Gain3/1 -> Gain16/1
  Gain16/1 -> Sum7/2
  Gain2/1 -> Gain17/1
  Gain17/1 -> Sum7/1
  Gain18/1 -> Sum5/1
  Gain19/1 -> Sum9/1
  Gain20/1 -> Sum9/2
  Sum6/1 -> Gain7/1
  Gain23/1 -> Sum5/2
  Sum8/1 -> Gain3/1
  Bus Selector7/3 -> phi adjust/1  "<phi>"
  Saturation2/1 -> Gain21/1
  Gain24/1 -> Sum11/1
  Gain25/1 -> Sum11/2
  Gain26/1 -> Saturation4/1
  Bus Selector7/1 -> Sum21/2  "<y>"
  Gain29/1 -> Sum22/1
  Gain15/1 -> Sum18/1
  Gain21/1 -> torquetheta/1
  Fcn4/1 -> Bus Creator/1  "xr"
  theta adjust/1 -> Sum8/2
  phi adjust/1 -> Sum6/2
  theta dot adjust/1 -> Sum19/2
  phi dot adjust/1 -> Sum24/2
  Saturation4/1 -> torquepsi/1

== system imageSendExample2/Controller/Conversion torques to motor speeds ==
  torques and thrust : Inport
  MATLAB Function : MATLAB Function  TreatAsAtomicUnit=on
  MATLAB Function1 : Subsystem  Commented=on  TreatAsAtomicUnit=on
  forcestorques2motorspeeds : MATLABFcn  Commented=on  MATLABFcn=forcestorques2motorspeeds  OutputDimensions=4
  Motor speeds : Outport
  wires:
  MATLAB Function/1(y) -> Motor speeds/1
  torques and thrust/1 -> MATLAB Function/1(u)

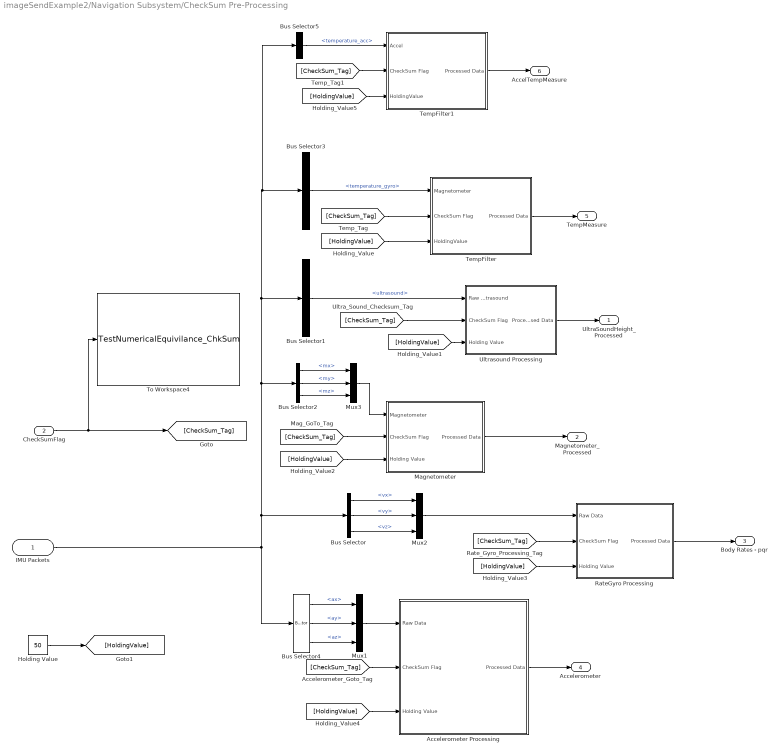
== system imageSendExample2/Navigation Subsystem/CheckSum Pre-Processing ==
  IMU Packets : Inport
  CheckSumFlag : Inport  Port=2
  Accelerometer Processing : Subsystem
  Bus Selector : BusSelector  OutputSignals=vx,vy,vz
  Bus Selector1 : BusSelector  OutputSignals=ultrasound
  Bus Selector2 : BusSelector  OutputSignals=mx,my,mz
  Bus Selector3 : BusSelector  OutputSignals=temperature_gyro
  Bus Selector4 : BusSelector  OutputSignals=ax,ay,az
  Bus Selector5 : BusSelector  OutputSignals=temperature_acc
  Holding Value : Constant  Value=50
  Magnetometer : Subsystem
  Mux1 : Mux  Inputs=3
  Mux2 : Mux  Inputs=3
  Mux3 : Mux  Inputs=3
  RateGyro Processing : Subsystem
  TempFilter : Subsystem
  TempFilter1 : Subsystem
  To Workspace4 : ToWorkspace  VariableName=TestNumericalEquivilance_ChkSum  SaveFormat=Structure With Time  SampleTime=-1
  Ultrasound Processing : Subsystem
  UltraSoundHeight_Processed : Outport
  Magnetometer_Processed : Outport  Port=2
  Body Rates - pqr : Outport  Port=3
  Accelerometer : Outport  Port=4
  TempMeasure : Outport  Port=5
  AccelTempMeasure : Outport  Port=6
  wires:
  Bus Selector1/1 -> Ultrasound Processing/1(Raw Ultrasound)  "<ultrasound>"
  CheckSumFlag/1 -> To Workspace4/1, [CheckSum_Tag]
  IMU Packets/1 -> Bus Selector/1, Bus Selector5/1, Bus Selector3/1, Bus Selector1/1, Bus Selector2/1, Bus Selector4/1
  Bus Selector4/1 -> Mux1/1  "<ax>"
  Bus Selector4/2 -> Mux1/2  "<ay>"
  Bus Selector4/3 -> Mux1/3  "<az>"
  Mux1/1 -> Accelerometer Processing/1(Raw Data)
  [CheckSum_Tag] -> Ultrasound Processing/2(CheckSum Flag)
  Accelerometer Processing/1(Processed Data) -> Accelerometer/1
  Mux2/1 -> RateGyro Processing/1(Raw Data)
  [CheckSum_Tag] -> RateGyro Processing/2(CheckSum Flag)
  RateGyro Processing/1(Processed Data) -> Body Rates - pqr/1
  Bus Selector2/1 -> Mux3/1  "<mx>"
  Bus Selector2/2 -> Mux3/2  "<my>"
  Bus Selector2/3 -> Mux3/3  "<mz>"
  [CheckSum_Tag] -> Magnetometer/2(CheckSum Flag)
  Magnetometer/1(Processed Data) -> Magnetometer_Processed/1
  [CheckSum_Tag] -> Accelerometer Processing/2(CheckSum Flag)
  Ultrasound Processing/1(Processed Data) -> UltraSoundHeight_Processed/1
  Bus Selector/1 -> Mux2/1  "<vx>"
  Bus Selector/2 -> Mux2/2  "<vy>"
  Bus Selector/3 -> Mux2/3  "<vz>"
  Bus Selector3/1 -> TempFilter/1(Magnetometer)  "<temperature_gyro>"
  TempFilter/1(Processed Data) -> TempMeasure/1
  [CheckSum_Tag] -> TempFilter/2(CheckSum Flag)
  [HoldingValue] -> TempFilter/3(HoldingValue)
  [HoldingValue] -> Ultrasound Processing/3(Holding Value)
  [HoldingValue] -> Magnetometer/3(Holding Value)
  [HoldingValue] -> RateGyro Processing/3(Holding Value)
  [HoldingValue] -> Accelerometer Processing/3(Holding Value)
  Holding Value/1 -> [HoldingValue]
  Mux3/1 -> Magnetometer/1(Magnetometer)
  TempFilter1/1(Processed Data) -> AccelTempMeasure/1
  [CheckSum_Tag] -> TempFilter1/2(CheckSum Flag)
  [HoldingValue] -> TempFilter1/3(HoldingValue)
  Bus Selector5/1 -> TempFilter1/1(Accel)  "<temperature_acc>"

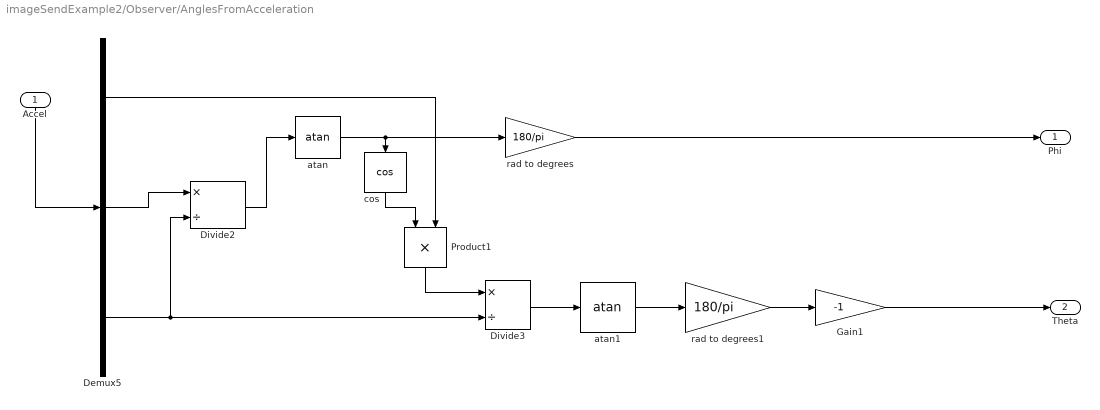
== system imageSendExample2/Observer/AnglesFromAcceleration ==
  Accel : Inport
  Demux5 : Demux  Outputs=3
  Divide2 : Product  Inputs=*/
  Divide3 : Product  Inputs=*/
  Gain1 : Gain  Gain=-1
  Product1 : Product
  atan : Trigonometry  Operator=atan
  atan1 : Trigonometry  Operator=atan
  cos : Trigonometry  Operator=cos
  rad to degrees : Gain  Gain=180/pi
  rad to degrees1 : Gain  Gain=180/pi
  Phi : Outport
  Theta : Outport  Port=2
  wires:
  Accel/1 -> Demux5/1
  Divide2/1 -> atan/1
  cos/1 -> Product1/1
  Demux5/2 -> Divide2/1
  Gain1/1 -> Theta/1
  rad to degrees/1 -> Phi/1
  Demux5/1 -> Product1/2
  Divide3/1 -> atan1/1
  atan1/1 -> rad to degrees1/1
  atan/1 -> rad to degrees/1, cos/1
  rad to degrees1/1 -> Gain1/1
  Demux5/3 -> Divide2/2, Divide3/2
  Product1/1 -> Divide3/1

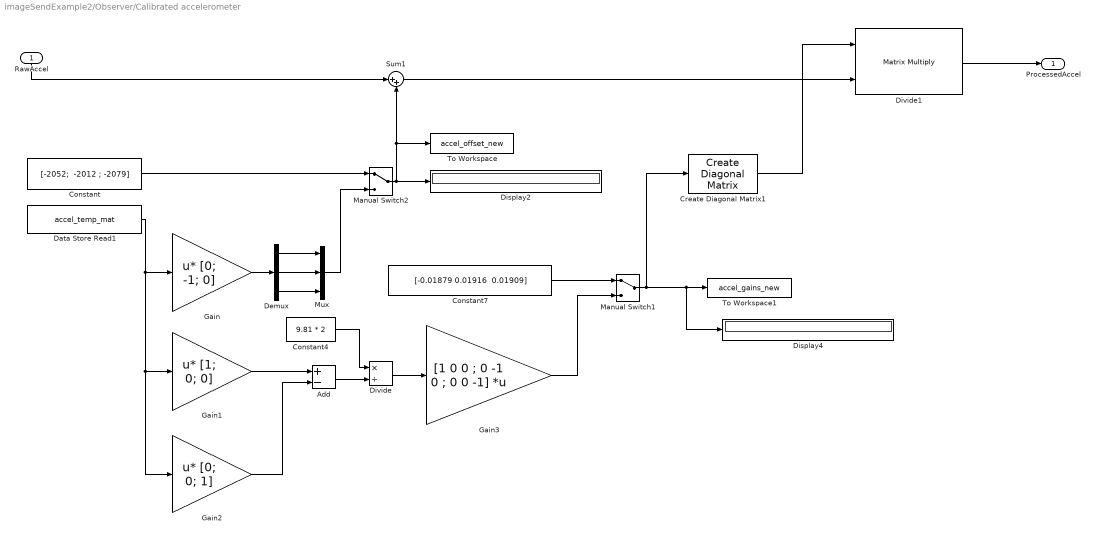
== system imageSendExample2/Observer/Calibrated accelerometer ==
  RawAccel : Inport
  Add : Sum  Inputs=+-
  Constant : Constant  Value="[-2052;  -2012 ; -2079]"
  Constant4 : Constant  Value=9.81 * 2
  Constant7 : Constant  Value="[-0.01879 0.01916  0.01909]"
  Create Diagonal Matrix1 : dspmtrx3/Create Diagonal Matrix
  Data Store Read1 : DataStoreRead  DataStoreName=accel_temp_mat
  Demux : Demux  Outputs=3
  Display2 : Display
  Display4 : Display
  Divide : Product  Inputs=*/
  Divide1 : Product  Inputs=**  Multiplication=Matrix(*)
  Gain : Gain  Gain="[0;  -1;  0]"  Multiplication=Matrix(u*K)
  Gain1 : Gain  Gain="[1;  0;  0]"  Multiplication=Matrix(u*K)
  Gain2 : Gain  Gain="[0;  0;  1]"  Multiplication=Matrix(u*K)
  Gain3 : Gain  Gain=[1 0 0 ; 0 -1 0 ; 0 0 -1]  Multiplication=Matrix(K*u)
  Manual Switch1 : ManualSwitch
  Manual Switch2 : ManualSwitch
  Mux : Mux  Inputs=3
  Sum1 : Sum  Inputs=|++
  To Workspace : ToWorkspace  VariableName=accel_offset_new  SaveFormat=Timeseries  SampleTime=-1
  To Workspace1 : ToWorkspace  VariableName=accel_gains_new  SaveFormat=Timeseries  SampleTime=-1
  ProcessedAccel : Outport
  wires:
  Sum1/1 -> Divide1/2
  Divide1/1 -> ProcessedAccel/1
  RawAccel/1 -> Sum1/1
  Constant/1 -> Manual Switch2/1
  Manual Switch2/1 -> To Workspace/1, Sum1/2, Display2/1
  Data Store Read1/1 -> Gain2/1, Gain1/1, Gain/1
  Gain1/1 -> Add/1
  Divide/1 -> Gain3/1
  Add/1 -> Divide/2
  Constant4/1 -> Divide/1
  Manual Switch1/1 -> Display4/1, To Workspace1/1, Create Diagonal Matrix1/1
  Gain3/1 -> Manual Switch1/2
  Create Diagonal Matrix1/1 -> Divide1/1
  Constant7/1 -> Manual Switch1/1
  Demux/1 -> Mux/1
  Demux/2 -> Mux/2
  Demux/3 -> Mux/3
  Gain/1 -> Demux/1
  Mux/1 -> Manual Switch2/2
  Gain2/1 -> Add/2

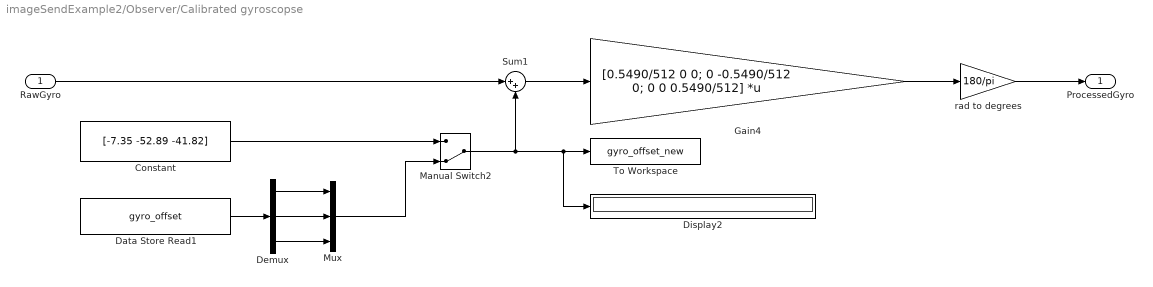
== system imageSendExample2/Observer/Calibrated gyroscopse ==
  RawGyro : Inport
  Constant : Constant  Value=[-7.35 -52.89 -41.82]
  Data Store Read1 : DataStoreRead  DataStoreName=gyro_offset
  Demux : Demux  Outputs=3
  Display2 : Display
  Gain4 : Gain  Gain=[0.5490/512 0 0; 0 -0.5490/512 0; 0 0 0.5490/512]  Multiplication=Matrix(K*u) (u vector)
  Manual Switch2 : ManualSwitch  CurrentSetting=0
  Mux : Mux  Inputs=3
  Sum1 : Sum  Inputs=|++
  To Workspace : ToWorkspace  VariableName=gyro_offset_new  SaveFormat=Timeseries  SampleTime=-1
  rad to degrees : Gain  Gain=180/pi
  ProcessedGyro : Outport
  wires:
  Gain4/1 -> rad to degrees/1
  Sum1/1 -> Gain4/1
  RawGyro/1 -> Sum1/1
  Constant/1 -> Manual Switch2/1
  Manual Switch2/1 -> Display2/1, To Workspace/1, Sum1/2
  Data Store Read1/1 -> Demux/1
  Mux/1 -> Manual Switch2/2
  Demux/1 -> Mux/1
  Demux/2 -> Mux/2
  Demux/3 -> Mux/3
  rad to degrees/1 -> ProcessedGyro/1

== system imageSendExample2/Controller/Conversion torques to motor speeds/MATLAB Function1 ==
  forcestorques : Inport
  " Demux " : Demux  Outputs=1
  " SFunction " : S-Function  Tag=Stateflow S-Function simQuad1 1  FunctionName=sf_sfun  PortCounts=[1 2]  EnableBusSupport=on
  " Terminator " : Terminator
  motorspeeds : Outport
  wires:
  forcestorques/1 -> " SFunction "/1
  " SFunction "/2 -> motorspeeds/1  "motorspeeds"
  " Demux "/1 -> " Terminator "/1
  " SFunction "/1 -> " Demux "/1

== system imageSendExample2/Navigation Subsystem/CheckSum Pre-Processing/Accelerometer Processing ==
  Raw Data : Inport
  CheckSum Flag : Inport  Port=2
  Holding Value : Inport  Port=3
  Calculate Accel Data : Subsystem  Commented=through
  CheckSum Correction : Subsystem
  Processed Data : Outport
  wires:
  CheckSum Flag/1 -> CheckSum Correction/2(CheckSumFlag)
  Raw Data/1 -> Calculate Accel Data/1(Raw Accel Data)
  CheckSum Correction/1(Pre-Processed Height) -> Processed Data/1
  Calculate Accel Data/1(Processed Accel Data) -> CheckSum Correction/1(CalculatedData)
  Holding Value/1 -> CheckSum Correction/3(Holding Value)

== system imageSendExample2/Navigation Subsystem/CheckSum Pre-Processing/Magnetometer ==
  Magnetometer : Inport
  CheckSum Flag : Inport  Port=2
  Holding Value : Inport  Port=3
  CheckSum Correction : Subsystem
  Process Raw Mag Data : Subsystem  Commented=through
  Processed Data : Outport
  wires:
  CheckSum Flag/1 -> CheckSum Correction/2(CheckSumFlag)
  CheckSum Correction/1(Pre-Processed Data) -> Processed Data/1
  Magnetometer/1 -> Process Raw Mag Data/1(Magnetometer)
  Process Raw Mag Data/1(ProcessedData) -> CheckSum Correction/1(CalculatedData)
  Holding Value/1 -> CheckSum Correction/3(Holding Value)

== system imageSendExample2/Navigation Subsystem/CheckSum Pre-Processing/RateGyro Processing ==
  Raw Data : Inport
  CheckSum Flag : Inport  Port=2
  Holding Value : Inport  Port=3
  CheckSum Correction : Subsystem
  Process Data : Subsystem  Commented=through
  Processed Data : Outport
  wires:
  CheckSum Flag/1 -> CheckSum Correction/2(CheckSumFlag)
  CheckSum Correction/1(Pre-Processed Height) -> Processed Data/1
  Raw Data/1 -> Process Data/1(Raw Data)
  Process Data/1(Processed Data) -> CheckSum Correction/1(CalculatedData)
  Holding Value/1 -> CheckSum Correction/3(Holding Value)

== system imageSendExample2/Navigation Subsystem/CheckSum Pre-Processing/TempFilter ==
  Magnetometer : Inport
  CheckSum Flag : Inport  Port=2
  HoldingValue : Inport  Port=3
  CheckSum Correction : Subsystem
  Process Raw Mag Data : Subsystem  Commented=through
  Processed Data : Outport
  wires:
  CheckSum Flag/1 -> CheckSum Correction/2(CheckSumFlag)
  CheckSum Correction/1(Pre-Processed Data) -> Processed Data/1
  Magnetometer/1 -> Process Raw Mag Data/1(Magnetometer)
  Process Raw Mag Data/1(ProcessedData) -> CheckSum Correction/1(CalculatedData)
  HoldingValue/1 -> CheckSum Correction/3(Holding Value)

== system imageSendExample2/Navigation Subsystem/CheckSum Pre-Processing/TempFilter1 ==
  Accel : Inport
  CheckSum Flag : Inport  Port=2
  HoldingValue : Inport  Port=3
  CheckSum Correction : Subsystem
  Process Raw Mag Data : Subsystem  Commented=through
  Processed Data : Outport
  wires:
  CheckSum Flag/1 -> CheckSum Correction/2(CheckSumFlag)
  CheckSum Correction/1(Pre-Processed Data) -> Processed Data/1
  Accel/1 -> Process Raw Mag Data/1(Magnetometer)
  Process Raw Mag Data/1(ProcessedData) -> CheckSum Correction/1(CalculatedData)
  HoldingValue/1 -> CheckSum Correction/3(Holding Value)

== system imageSendExample2/Navigation Subsystem/CheckSum Pre-Processing/Ultrasound Processing ==
  note: '192.168.1.1' 1 17725
  Raw Ultrasound : Inport
  CheckSum Flag : Inport  Port=2
  Holding Value : Inport  Port=3
  CheckSum Correction : Subsystem
  Data Type Conversion1 : DataTypeConversion
  Delay1 : Delay  DelayLength=1  InitialCondition=0
  Height Calculation : MATLAB Function  TreatAsAtomicUnit=on
  Saturation1 : Saturate  UpperLimit=100e3  LowerLimit=0
  Processed Data : Outport
  wires:
  Delay1/1 -> Height Calculation/2(z_1)
  Data Type Conversion1/1 -> Height Calculation/1(u)
  Height Calculation/2(prev_good_height) -> Delay1/1
  Raw Ultrasound/1 -> Data Type Conversion1/1
  Height Calculation/1(y) -> CheckSum Correction/1(CalculatedData)
  CheckSum Flag/1 -> CheckSum Correction/2(CheckSumFlag)
  CheckSum Correction/1(Pre-Processed Height) -> Saturation1/1
  Saturation1/1 -> Processed Data/1
  Holding Value/1 -> CheckSum Correction/3(Holding Value)

== system imageSendExample2/Navigation Subsystem/CheckSum Pre-Processing/Accelerometer Processing/Calculate Accel Data ==
  Raw Accel Data : Inport
  Bias : Constant  Value=[0 4096 4096]
  Gain : Gain  Gain=[0.001953125, 0.001953125, 0.001953125]
  Neutral Bias : Constant  Value=[2048 2048 2048]
  Sum : Sum  Inputs=|-+
  Sum1 : Sum  Inputs=|+-
  Processed Accel Data : Outport
  wires:
  Raw Accel Data/1 -> Sum/1
  Sum1/1 -> Gain/1
  Gain/1 -> Processed Accel Data/1
  Sum/1 -> Sum1/1
  Neutral Bias/1 -> Sum1/2
  Bias/1 -> Sum/2

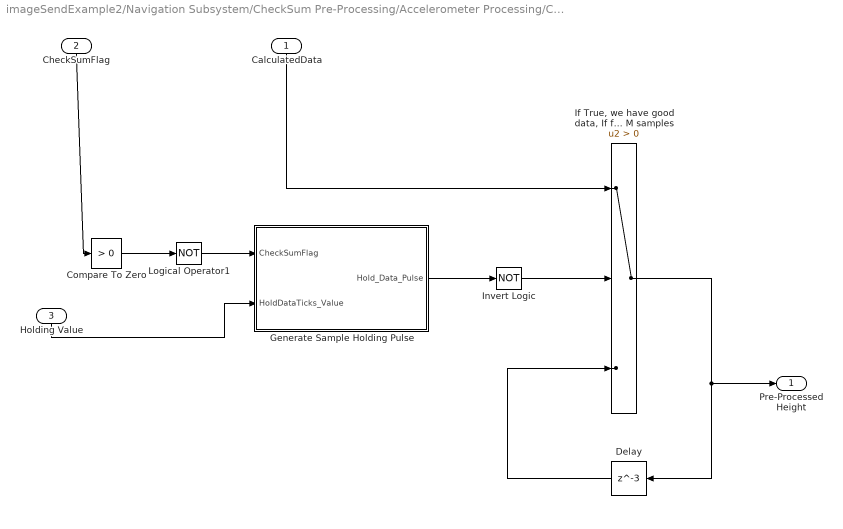
== system imageSendExample2/Navigation Subsystem/CheckSum Pre-Processing/Accelerometer Processing/CheckSum Correction ==
  CalculatedData : Inport
  CheckSumFlag : Inport  Port=2
  Holding Value : Inport  Port=3
  Compare To Zero : simulink/Logic and Bit Operations/Compare To Zero  relop=>  OutDataTypeStr=boolean
  Delay : Delay  DelayLength=3  InitialCondition=0
  Generate Sample Holding Pulse : Subsystem
  "If True, we have good data, If false, we have bad data, With bad data, use previous good data from N samples ago and hold it on that value for M samples" : Switch  Criteria=u2 > Threshold
  Invert Logic : Logic  Operator=NOT  AllPortsSameDT=off  OutDataTypeStr=boolean
  Logical Operator1 : Logic  Operator=NOT  AllPortsSameDT=off  OutDataTypeStr=boolean
  Pre-Processed Height : Outport
  wires:
  CheckSumFlag/1 -> Compare To Zero/1
  CalculatedData/1 -> "If True, we have good data, If false, we have bad data, With bad data, use previous good data from N samples ago and hold it on that value for M samples"/1
  "If True, we have good data, If false, we have bad data, With bad data, use previous good data from N samples ago and hold it on that value for M samples"/1 -> Pre-Processed Height/1, Delay/1
  Delay/1 -> "If True, we have good data, If false, we have bad data, With bad data, use previous good data from N samples ago and hold it on that value for M samples"/3
  Compare To Zero/1 -> Logical Operator1/1
  Generate Sample Holding Pulse/1(Hold_Data_Pulse) -> Invert Logic/1
  Logical Operator1/1 -> Generate Sample Holding Pulse/1(CheckSumFlag)
  Invert Logic/1 -> "If True, we have good data, If false, we have bad data, With bad data, use previous good data from N samples ago and hold it on that value for M samples"/2
  Holding Value/1 -> Generate Sample Holding Pulse/2(HoldDataTicks_Value)

== system imageSendExample2/Navigation Subsystem/CheckSum Pre-Processing/Magnetometer/CheckSum Correction ==
  CalculatedData : Inport
  CheckSumFlag : Inport  Port=2
  Holding Value : Inport  Port=3
  Compare To Zero : simulink/Logic and Bit Operations/Compare To Zero  relop=>  OutDataTypeStr=boolean
  Delay : Delay  DelayLength=3  InitialCondition=0
  Generate Sample Holding Pulse : Subsystem
  "If True, we have good data, If false, we have bad data, With bad data, use previous good data from N samples ago and hold it on that value for M samples" : Switch  Criteria=u2 > Threshold
  Invert Logic : Logic  Operator=NOT  AllPortsSameDT=off  OutDataTypeStr=boolean
  Logical Operator1 : Logic  Operator=NOT  AllPortsSameDT=off  OutDataTypeStr=boolean
  Pre-Processed Data : Outport
  wires:
  CheckSumFlag/1 -> Compare To Zero/1
  CalculatedData/1 -> "If True, we have good data, If false, we have bad data, With bad data, use previous good data from N samples ago and hold it on that value for M samples"/1
  "If True, we have good data, If false, we have bad data, With bad data, use previous good data from N samples ago and hold it on that value for M samples"/1 -> Pre-Processed Data/1, Delay/1
  Delay/1 -> "If True, we have good data, If false, we have bad data, With bad data, use previous good data from N samples ago and hold it on that value for M samples"/3
  Compare To Zero/1 -> Logical Operator1/1
  Generate Sample Holding Pulse/1(Hold_Data_Pulse) -> Invert Logic/1
  Logical Operator1/1 -> Generate Sample Holding Pulse/1(CheckSumFlag)
  Invert Logic/1 -> "If True, we have good data, If false, we have bad data, With bad data, use previous good data from N samples ago and hold it on that value for M samples"/2
  Holding Value/1 -> Generate Sample Holding Pulse/2(HoldDataTicks_Value)

== system imageSendExample2/Navigation Subsystem/CheckSum Pre-Processing/Magnetometer/Process Raw Mag Data ==
  note: magnetometer[ 0 ] = - ( float ) navdata.mx ;
      | magnetometer[ 1 ] = ( float ) navdata.my ;
      | magnetometer[ 2 ] = - ( float ) navdata.mz ;
      | const float Sensitivity[ 3 ] = { 0.0071492608 , 0.0070882491 , 0.0074057781 } ;
      | const float Neutral[ 3 ] = { 118.0 , - 65.0 , 110.0 } ;
  Magnetometer : Inport
  Bias : Constant  Value=[ 118.0, -65.0, 110.0 ]
  Sum : Sum  Inputs=|+-
  postGain : Gain  Gain=[0.0071492608, 0.0070882491, 0.0074057781]
  preGain : Gain  Gain=[-1 1 -1]
  ProcessedData : Outport
  wires:
  postGain/1 -> ProcessedData/1
  Magnetometer/1 -> preGain/1
  Sum/1 -> postGain/1
  preGain/1 -> Sum/1
  Bias/1 -> Sum/2

== system imageSendExample2/Navigation Subsystem/CheckSum Pre-Processing/RateGyro Processing/CheckSum Correction ==
  CalculatedData : Inport
  CheckSumFlag : Inport  Port=2
  Holding Value : Inport  Port=3
  Compare To Zero : simulink/Logic and Bit Operations/Compare To Zero  relop=>  OutDataTypeStr=boolean
  Delay : Delay  DelayLength=3  InitialCondition=0
  Generate Sample Holding Pulse : Subsystem
  "If True, we have good data, If false, we have bad data, With bad data, use previous good data from N samples ago and hold it on that value for M samples" : Switch  Criteria=u2 > Threshold
  Invert Logic : Logic  Operator=NOT  AllPortsSameDT=off  OutDataTypeStr=boolean
  Logical Operator1 : Logic  Operator=NOT  AllPortsSameDT=off  OutDataTypeStr=boolean
  Pre-Processed Height : Outport
  wires:
  CheckSumFlag/1 -> Compare To Zero/1
  CalculatedData/1 -> "If True, we have good data, If false, we have bad data, With bad data, use previous good data from N samples ago and hold it on that value for M samples"/1
  "If True, we have good data, If false, we have bad data, With bad data, use previous good data from N samples ago and hold it on that value for M samples"/1 -> Pre-Processed Height/1, Delay/1
  Delay/1 -> "If True, we have good data, If false, we have bad data, With bad data, use previous good data from N samples ago and hold it on that value for M samples"/3
  Compare To Zero/1 -> Logical Operator1/1
  Generate Sample Holding Pulse/1(Hold_Data_Pulse) -> Invert Logic/1
  Logical Operator1/1 -> Generate Sample Holding Pulse/1(CheckSumFlag)
  Invert Logic/1 -> "If True, we have good data, If false, we have bad data, With bad data, use previous good data from N samples ago and hold it on that value for M samples"/2
  Holding Value/1 -> Generate Sample Holding Pulse/2(HoldDataTicks_Value)

== system imageSendExample2/Navigation Subsystem/CheckSum Pre-Processing/RateGyro Processing/Process Data ==
  note: const float Sensitivity[ 3 ] = { 0.0609 , 0.0609 , 0.0609 } ;
      | const float Neutral[ 3 ] = { 0.0 , 0.0 , 0.0 } ;
      | const int16_t Offset[ 3 ] = { - 73 , 14 , - 13 } ;
      | const int16_t Noises[ 3 ] = { 35 , 35 , 15 } ;
      |
      | int16_t vRaws[ 3 ] = {
      | Navdata :: IMU :: Gyroscope :: getRawX (),
      | Navdata :: IMU :: Gyroscope :: getRawY (),
      | Navdata :: IMU :: Gyroscope :: getRawZ ()
      | } ;
      |
      | gyroscope[i] = vRaws[i] * Gyroscope :: Sensitivity[i] * M_PI / 180.0 ;
  Raw Data : Inport
  Constant : Constant  Value=[0.0, 0.0, 0.0]
  Gain : Gain  Gain=[0.0609, 0.0609, 0.0609]
  Sum : Sum  Inputs=|++
  Processed Data : Outport
  wires:
  Sum/1 -> Gain/1
  Gain/1 -> Processed Data/1
  Constant/1 -> Sum/2
  Raw Data/1 -> Sum/1
